simulink model "Model_with_decision"  (R2022a)
settings: Solver=VariableStepAuto  StartTime=0.0  StopTime=1000000  RelTol=1e-3
undefined symbols (not defined in the file): Coefficient_value, Enable_X, Enable_Y, N, s1, s10, s11, s12, s13, s14, s15, s16, s17, s18, s19, s2, s20, s21, s22, s23, s24, s25, s26, s27, s28, s29, s3, s30, s4, s5, s6, s7, s8, s9
libraries: simulink x35
(part 5 of 5)

== system Model_with_decision/Pbit_2/EN=1 Block ==
  note: this is boolean
  note: threshold is subtracted from the sum of total input and random value to implement > 1 comparison
  IN : Inport
  Action Port : ActionPort  ActionPortLabel=if(u1 > 0)
  Add : Sum
  Add1 : Sum
  Compare To Constant : simulink/Logic and Bit Operations/Compare To Constant  relop=>  const=1  OutDataTypeStr=boolean
  Constant : Constant  Value=-1
  Constant1 : Constant
  Constant2 : Constant
  Divide : Product  Inputs=*/
  Math Function : Math
  Product : Product
  Uniform Random Number : UniformRandomNumber  Minimum=0  Seed=s2  SampleTime=1
  OUT : Outport
  wires:
  Add1/1 -> Divide/2
  Constant2/1 -> Divide/1
  Math Function/1 -> Add1/1
  Product/1 -> Math Function/1
  Constant1/1 -> Add1/2
  Constant/1 -> Product/2
  Divide/1 -> Add/1
  IN/1 -> Product/1
  Compare To Constant/1 -> OUT/1
  Add/1 -> Compare To Constant/1
  Uniform Random Number/1 -> Add/2

== system Model_with_decision/Pbit_3/EN=0 Block ==
  IN : Inport
  Action Port : ActionPort  ActionPortLabel=else
  Out1 : Outport
  wires:
  IN/1 -> Out1/1

== system Model_with_decision/Pbit_3/EN=1 Block ==
  note: threshold is subtracted from the sum of total input and random value to implement > 1 comparison
  note: this is boolean
  IN : Inport
  Action Port : ActionPort  ActionPortLabel=if(u1 > 0)
  Add : Sum
  Add1 : Sum
  Compare To Constant : simulink/Logic and Bit Operations/Compare To Constant  relop=>  const=1  OutDataTypeStr=boolean
  Constant : Constant  Value=-1
  Constant1 : Constant
  Constant2 : Constant
  Divide : Product  Inputs=*/
  Math Function : Math
  Product : Product
  Uniform Random Number : UniformRandomNumber  Minimum=0  Seed=s3  SampleTime=1
  OUT : Outport
  wires:
  Uniform Random Number/1 -> Add/2
  Add/1 -> Compare To Constant/1
  Compare To Constant/1 -> OUT/1
  IN/1 -> Product/1
  Divide/1 -> Add/1
  Constant/1 -> Product/2
  Constant1/1 -> Add1/2
  Product/1 -> Math Function/1
  Math Function/1 -> Add1/1
  Constant2/1 -> Divide/1
  Add1/1 -> Divide/2

== system Model_with_decision/Pbit_4/EN=0 Block ==
  IN : Inport
  Action Port : ActionPort  ActionPortLabel=else
  Out1 : Outport
  wires:
  IN/1 -> Out1/1

== system Model_with_decision/Pbit_4/EN=1 Block ==
  note: threshold is subtracted from the sum of total input and random value to implement > 1 comparison
  note: this is boolean
  IN : Inport
  Action Port : ActionPort  ActionPortLabel=if(u1 > 0)
  Add : Sum
  Add1 : Sum
  Compare To Constant : simulink/Logic and Bit Operations/Compare To Constant  relop=>  const=1  OutDataTypeStr=boolean
  Constant : Constant  Value=-1
  Constant1 : Constant
  Constant2 : Constant
  Divide : Product  Inputs=*/
  Math Function : Math
  Product : Product
  Uniform Random Number : UniformRandomNumber  Minimum=0  Seed=s4  SampleTime=1
  OUT : Outport
  wires:
  Uniform Random Number/1 -> Add/2
  Add/1 -> Compare To Constant/1
  Compare To Constant/1 -> OUT/1
  IN/1 -> Product/1
  Divide/1 -> Add/1
  Constant/1 -> Product/2
  Constant1/1 -> Add1/2
  Product/1 -> Math Function/1
  Math Function/1 -> Add1/1
  Constant2/1 -> Divide/1
  Add1/1 -> Divide/2

== system Model_with_decision/Pbit_5/EN=0 Block ==
  IN : Inport
  Action Port : ActionPort  ActionPortLabel=else
  Out1 : Outport
  wires:
  IN/1 -> Out1/1

== system Model_with_decision/Pbit_5/EN=1 Block ==
  note: this is boolean
  note: threshold is subtracted from the sum of total input and random value to implement > 1 comparison
  IN : Inport
  Action Port : ActionPort  ActionPortLabel=if(u1 > 0)
  Add : Sum
  Add1 : Sum
  Compare To Constant : simulink/Logic and Bit Operations/Compare To Constant  relop=>  const=1  OutDataTypeStr=boolean
  Constant : Constant  Value=-1
  Constant1 : Constant
  Constant2 : Constant
  Divide : Product  Inputs=*/
  Math Function : Math
  Product : Product
  Uniform Random Number : UniformRandomNumber  Minimum=0  Seed=s5  SampleTime=1
  OUT : Outport
  wires:
  Add1/1 -> Divide/2
  Constant2/1 -> Divide/1
  Math Function/1 -> Add1/1
  Product/1 -> Math Function/1
  Constant1/1 -> Add1/2
  Constant/1 -> Product/2
  Divide/1 -> Add/1
  IN/1 -> Product/1
  Compare To Constant/1 -> OUT/1
  Add/1 -> Compare To Constant/1
  Uniform Random Number/1 -> Add/2

== system Model_with_decision/Pbit_6/EN=0 Block ==
  IN : Inport
  Action Port : ActionPort  ActionPortLabel=else
  Out1 : Outport
  wires:
  IN/1 -> Out1/1

== system Model_with_decision/Pbit_6/EN=1 Block ==
  note: this is boolean
  note: threshold is subtracted from the sum of total input and random value to implement > 1 comparison
  IN : Inport
  Action Port : ActionPort  ActionPortLabel=if(u1 > 0)
  Add : Sum
  Add1 : Sum
  Compare To Constant : simulink/Logic and Bit Operations/Compare To Constant  relop=>  const=1  OutDataTypeStr=boolean
  Constant : Constant  Value=-1
  Constant1 : Constant
  Constant2 : Constant
  Divide : Product  Inputs=*/
  Math Function : Math
  Product : Product
  Uniform Random Number : UniformRandomNumber  Minimum=0  Seed=s6  SampleTime=1
  OUT : Outport
  wires:
  Add1/1 -> Divide/2
  Constant2/1 -> Divide/1
  Math Function/1 -> Add1/1
  Product/1 -> Math Function/1
  Constant1/1 -> Add1/2
  Constant/1 -> Product/2
  Divide/1 -> Add/1
  IN/1 -> Product/1
  Compare To Constant/1 -> OUT/1
  Add/1 -> Compare To Constant/1
  Uniform Random Number/1 -> Add/2

== system Model_with_decision/Pbit_7/EN=0 Block ==
  IN : Inport
  Action Port : ActionPort  ActionPortLabel=else
  Out1 : Outport
  wires:
  IN/1 -> Out1/1

== system Model_with_decision/Pbit_7/EN=1 Block ==
  note: this is boolean
  note: threshold is subtracted from the sum of total input and random value to implement > 1 comparison
  IN : Inport
  Action Port : ActionPort  ActionPortLabel=if(u1 > 0)
  Add : Sum
  Add1 : Sum
  Compare To Constant : simulink/Logic and Bit Operations/Compare To Constant  relop=>  const=1  OutDataTypeStr=boolean
  Constant : Constant  Value=-1
  Constant1 : Constant
  Constant2 : Constant
  Divide : Product  Inputs=*/
  Math Function : Math
  Product : Product
  Uniform Random Number : UniformRandomNumber  Minimum=0  Seed=s7  SampleTime=1
  OUT : Outport
  wires:
  Add1/1 -> Divide/2
  Constant2/1 -> Divide/1
  Math Function/1 -> Add1/1
  Product/1 -> Math Function/1
  Constant1/1 -> Add1/2
  Constant/1 -> Product/2
  Divide/1 -> Add/1
  IN/1 -> Product/1
  Compare To Constant/1 -> OUT/1
  Add/1 -> Compare To Constant/1
  Uniform Random Number/1 -> Add/2

== system Model_with_decision/Pbit_8/EN=0 Block ==
  IN : Inport
  Action Port : ActionPort  ActionPortLabel=else
  Out1 : Outport
  wires:
  IN/1 -> Out1/1

== system Model_with_decision/Pbit_8/EN=1 Block ==
  note: threshold is subtracted from the sum of total input and random value to implement > 1 comparison
  note: this is boolean
  IN : Inport
  Action Port : ActionPort  ActionPortLabel=if(u1 > 0)
  Add : Sum
  Add1 : Sum
  Compare To Constant : simulink/Logic and Bit Operations/Compare To Constant  relop=>  const=1  OutDataTypeStr=boolean
  Constant : Constant  Value=-1
  Constant1 : Constant
  Constant2 : Constant
  Divide : Product  Inputs=*/
  Math Function : Math
  Product : Product
  Uniform Random Number : UniformRandomNumber  Minimum=0  Seed=s8  SampleTime=1
  OUT : Outport
  wires:
  Uniform Random Number/1 -> Add/2
  Add/1 -> Compare To Constant/1
  Compare To Constant/1 -> OUT/1
  IN/1 -> Product/1
  Divide/1 -> Add/1
  Constant/1 -> Product/2
  Constant1/1 -> Add1/2
  Product/1 -> Math Function/1
  Math Function/1 -> Add1/1
  Constant2/1 -> Divide/1
  Add1/1 -> Divide/2

== system Model_with_decision/Pbit_9/EN=0 Block ==
  IN : Inport
  Action Port : ActionPort  ActionPortLabel=else
  Out1 : Outport
  wires:
  IN/1 -> Out1/1

== system Model_with_decision/Pbit_9/EN=1 Block ==
  note: threshold is subtracted from the sum of total input and random value to implement > 1 comparison
  note: this is boolean
  IN : Inport
  Action Port : ActionPort  ActionPortLabel=if(u1 > 0)
  Add : Sum
  Add1 : Sum
  Compare To Constant : simulink/Logic and Bit Operations/Compare To Constant  relop=>  const=1  OutDataTypeStr=boolean
  Constant : Constant  Value=-1
  Constant1 : Constant
  Constant2 : Constant
  Divide : Product  Inputs=*/
  Math Function : Math
  Product : Product
  Uniform Random Number : UniformRandomNumber  Minimum=0  Seed=s9  SampleTime=1
  OUT : Outport
  wires:
  Uniform Random Number/1 -> Add/2
  Add/1 -> Compare To Constant/1
  Compare To Constant/1 -> OUT/1
  IN/1 -> Product/1
  Divide/1 -> Add/1
  Constant/1 -> Product/2
  Constant1/1 -> Add1/2
  Product/1 -> Math Function/1
  Math Function/1 -> Add1/1
  Constant2/1 -> Divide/1
  Add1/1 -> Divide/2

== system Model_with_decision/Pbit_Y_1/EN=0 Block ==
  IN : Inport
  Action Port : ActionPort  ActionPortLabel=else
  Out1 : Outport
  wires:
  IN/1 -> Out1/1

== system Model_with_decision/Pbit_Y_1/EN=1 Block ==
  note: this is boolean
  note: threshold is subtracted from the sum of total input and random value to implement > 1 comparison
  IN : Inport
  Action Port : ActionPort  ActionPortLabel=if(u1 > 0)
  Add : Sum
  Add1 : Sum
  Compare To Constant : simulink/Logic and Bit Operations/Compare To Constant  relop=>  const=1  OutDataTypeStr=boolean
  Constant : Constant  Value=-1
  Constant1 : Constant
  Constant2 : Constant
  Divide : Product  Inputs=*/
  Math Function : Math
  Product : Product
  Uniform Random Number : UniformRandomNumber  Minimum=0  Seed=s16  SampleTime=1
  OUT : Outport
  wires:
  Add1/1 -> Divide/2
  Constant2/1 -> Divide/1
  Math Function/1 -> Add1/1
  Product/1 -> Math Function/1
  Constant1/1 -> Add1/2
  Constant/1 -> Product/2
  Divide/1 -> Add/1
  IN/1 -> Product/1
  Compare To Constant/1 -> OUT/1
  Add/1 -> Compare To Constant/1
  Uniform Random Number/1 -> Add/2

== system Model_with_decision/Pbit_Y_10/EN=0 Block ==
  IN : Inport
  Action Port : ActionPort  ActionPortLabel=else
  Out1 : Outport
  wires:
  IN/1 -> Out1/1

== system Model_with_decision/Pbit_Y_10/EN=1 Block ==
  note: this is boolean
  note: threshold is subtracted from the sum of total input and random value to implement > 1 comparison
  IN : Inport
  Action Port : ActionPort  ActionPortLabel=if(u1 > 0)
  Add : Sum
  Add1 : Sum
  Compare To Constant : simulink/Logic and Bit Operations/Compare To Constant  relop=>  const=1  OutDataTypeStr=boolean
  Constant : Constant  Value=-1
  Constant1 : Constant
  Constant2 : Constant
  Divide : Product  Inputs=*/
  Math Function : Math
  Product : Product
  Uniform Random Number : UniformRandomNumber  Minimum=0  Seed=s25  SampleTime=1
  OUT : Outport
  wires:
  Add1/1 -> Divide/2
  Constant2/1 -> Divide/1
  Math Function/1 -> Add1/1
  Product/1 -> Math Function/1
  Constant1/1 -> Add1/2
  Constant/1 -> Product/2
  Divide/1 -> Add/1
  IN/1 -> Product/1
  Compare To Constant/1 -> OUT/1
  Add/1 -> Compare To Constant/1
  Uniform Random Number/1 -> Add/2

== system Model_with_decision/Pbit_Y_11/EN=0 Block ==
  IN : Inport
  Action Port : ActionPort  ActionPortLabel=else
  Out1 : Outport
  wires:
  IN/1 -> Out1/1

== system Model_with_decision/Pbit_Y_11/EN=1 Block ==
  note: this is boolean
  note: threshold is subtracted from the sum of total input and random value to implement > 1 comparison
  IN : Inport
  Action Port : ActionPort  ActionPortLabel=if(u1 > 0)
  Add : Sum
  Add1 : Sum
  Compare To Constant : simulink/Logic and Bit Operations/Compare To Constant  relop=>  const=1  OutDataTypeStr=boolean
  Constant : Constant  Value=-1
  Constant1 : Constant
  Constant2 : Constant
  Divide : Product  Inputs=*/
  Math Function : Math
  Product : Product
  Uniform Random Number : UniformRandomNumber  Minimum=0  Seed=s26  SampleTime=1
  OUT : Outport
  wires:
  Add1/1 -> Divide/2
  Constant2/1 -> Divide/1
  Math Function/1 -> Add1/1
  Product/1 -> Math Function/1
  Constant1/1 -> Add1/2
  Constant/1 -> Product/2
  Divide/1 -> Add/1
  IN/1 -> Product/1
  Compare To Constant/1 -> OUT/1
  Add/1 -> Compare To Constant/1
  Uniform Random Number/1 -> Add/2

== system Model_with_decision/Pbit_Y_12/EN=0 Block ==
  IN : Inport
  Action Port : ActionPort  ActionPortLabel=else
  Out1 : Outport
  wires:
  IN/1 -> Out1/1

== system Model_with_decision/Pbit_Y_12/EN=1 Block ==
  note: this is boolean
  note: threshold is subtracted from the sum of total input and random value to implement > 1 comparison
  IN : Inport
  Action Port : ActionPort  ActionPortLabel=if(u1 > 0)
  Add : Sum
  Add1 : Sum
  Compare To Constant : simulink/Logic and Bit Operations/Compare To Constant  relop=>  const=1  OutDataTypeStr=boolean
  Constant : Constant  Value=-1
  Constant1 : Constant
  Constant2 : Constant
  Divide : Product  Inputs=*/
  Math Function : Math
  Product : Product
  Uniform Random Number : UniformRandomNumber  Minimum=0  Seed=s27  SampleTime=1
  OUT : Outport
  wires:
  Add1/1 -> Divide/2
  Constant2/1 -> Divide/1
  Math Function/1 -> Add1/1
  Product/1 -> Math Function/1
  Constant1/1 -> Add1/2
  Constant/1 -> Product/2
  Divide/1 -> Add/1
  IN/1 -> Product/1
  Compare To Constant/1 -> OUT/1
  Add/1 -> Compare To Constant/1
  Uniform Random Number/1 -> Add/2

== system Model_with_decision/Pbit_Y_13/EN=0 Block ==
  IN : Inport
  Action Port : ActionPort  ActionPortLabel=else
  Out1 : Outport
  wires:
  IN/1 -> Out1/1

== system Model_with_decision/Pbit_Y_13/EN=1 Block ==
  note: threshold is subtracted from the sum of total input and random value to implement > 1 comparison
  note: this is boolean
  IN : Inport
  Action Port : ActionPort  ActionPortLabel=if(u1 > 0)
  Add : Sum
  Add1 : Sum
  Compare To Constant : simulink/Logic and Bit Operations/Compare To Constant  relop=>  const=1  OutDataTypeStr=boolean
  Constant : Constant  Value=-1
  Constant1 : Constant
  Constant2 : Constant
  Divide : Product  Inputs=*/
  Math Function : Math
  Product : Product
  Uniform Random Number : UniformRandomNumber  Minimum=0  Seed=s28  SampleTime=1
  OUT : Outport
  wires:
  Uniform Random Number/1 -> Add/2
  Add/1 -> Compare To Constant/1
  Compare To Constant/1 -> OUT/1
  IN/1 -> Product/1
  Divide/1 -> Add/1
  Constant/1 -> Product/2
  Constant1/1 -> Add1/2
  Product/1 -> Math Function/1
  Math Function/1 -> Add1/1
  Constant2/1 -> Divide/1
  Add1/1 -> Divide/2

== system Model_with_decision/Pbit_Y_14/EN=0 Block ==
  IN : Inport
  Action Port : ActionPort  ActionPortLabel=else
  Out1 : Outport
  wires:
  IN/1 -> Out1/1

== system Model_with_decision/Pbit_Y_14/EN=1 Block ==
  note: threshold is subtracted from the sum of total input and random value to implement > 1 comparison
  note: this is boolean
  IN : Inport
  Action Port : ActionPort  ActionPortLabel=if(u1 > 0)
  Add : Sum
  Add1 : Sum
  Compare To Constant : simulink/Logic and Bit Operations/Compare To Constant  relop=>  const=1  OutDataTypeStr=boolean
  Constant : Constant  Value=-1
  Constant1 : Constant
  Constant2 : Constant
  Divide : Product  Inputs=*/
  Math Function : Math
  Product : Product
  Uniform Random Number : UniformRandomNumber  Minimum=0  Seed=s29  SampleTime=1
  OUT : Outport
  wires:
  Uniform Random Number/1 -> Add/2
  Add/1 -> Compare To Constant/1
  Compare To Constant/1 -> OUT/1
  IN/1 -> Product/1
  Divide/1 -> Add/1
  Constant/1 -> Product/2
  Constant1/1 -> Add1/2
  Product/1 -> Math Function/1
  Math Function/1 -> Add1/1
  Constant2/1 -> Divide/1
  Add1/1 -> Divide/2

== system Model_with_decision/Pbit_Y_15/EN=0 Block ==
  IN : Inport
  Action Port : ActionPort  ActionPortLabel=else
  Out1 : Outport
  wires:
  IN/1 -> Out1/1

== system Model_with_decision/Pbit_Y_15/EN=1 Block ==
  note: threshold is subtracted from the sum of total input and random value to implement > 1 comparison
  note: this is boolean
  IN : Inport
  Action Port : ActionPort  ActionPortLabel=if(u1 > 0)
  Add : Sum
  Add1 : Sum
  Compare To Constant : simulink/Logic and Bit Operations/Compare To Constant  relop=>  const=1  OutDataTypeStr=boolean
  Constant : Constant  Value=-1
  Constant1 : Constant
  Constant2 : Constant
  Divide : Product  Inputs=*/
  Math Function : Math
  Product : Product
  Uniform Random Number : UniformRandomNumber  Minimum=0  Seed=s30  SampleTime=1
  OUT : Outport
  wires:
  Uniform Random Number/1 -> Add/2
  Add/1 -> Compare To Constant/1
  Compare To Constant/1 -> OUT/1
  IN/1 -> Product/1
  Divide/1 -> Add/1
  Constant/1 -> Product/2
  Constant1/1 -> Add1/2
  Product/1 -> Math Function/1
  Math Function/1 -> Add1/1
  Constant2/1 -> Divide/1
  Add1/1 -> Divide/2

== system Model_with_decision/Pbit_Y_2/EN=0 Block ==
  IN : Inport
  Action Port : ActionPort  ActionPortLabel=else
  Out1 : Outport
  wires:
  IN/1 -> Out1/1

== system Model_with_decision/Pbit_Y_2/EN=1 Block ==
  note: this is boolean
  note: threshold is subtracted from the sum of total input and random value to implement > 1 comparison
  IN : Inport
  Action Port : ActionPort  ActionPortLabel=if(u1 > 0)
  Add : Sum
  Add1 : Sum
  Compare To Constant : simulink/Logic and Bit Operations/Compare To Constant  relop=>  const=1  OutDataTypeStr=boolean
  Constant : Constant  Value=-1
  Constant1 : Constant
  Constant2 : Constant
  Divide : Product  Inputs=*/
  Math Function : Math
  Product : Product
  Uniform Random Number : UniformRandomNumber  Minimum=0  Seed=s17  SampleTime=1
  OUT : Outport
  wires:
  Add1/1 -> Divide/2
  Constant2/1 -> Divide/1
  Math Function/1 -> Add1/1
  Product/1 -> Math Function/1
  Constant1/1 -> Add1/2
  Constant/1 -> Product/2
  Divide/1 -> Add/1
  IN/1 -> Product/1
  Compare To Constant/1 -> OUT/1
  Add/1 -> Compare To Constant/1
  Uniform Random Number/1 -> Add/2

== system Model_with_decision/Pbit_Y_3/EN=0 Block ==
  IN : Inport
  Action Port : ActionPort  ActionPortLabel=else
  Out1 : Outport
  wires:
  IN/1 -> Out1/1

== system Model_with_decision/Pbit_Y_3/EN=1 Block ==
  note: threshold is subtracted from the sum of total input and random value to implement > 1 comparison
  note: this is boolean
  IN : Inport
  Action Port : ActionPort  ActionPortLabel=if(u1 > 0)
  Add : Sum
  Add1 : Sum
  Compare To Constant : simulink/Logic and Bit Operations/Compare To Constant  relop=>  const=1  OutDataTypeStr=boolean
  Constant : Constant  Value=-1
  Constant1 : Constant
  Constant2 : Constant
  Divide : Product  Inputs=*/
  Math Function : Math
  Product : Product
  Uniform Random Number : UniformRandomNumber  Minimum=0  Seed=s18  SampleTime=1
  OUT : Outport
  wires:
  Uniform Random Number/1 -> Add/2
  Add/1 -> Compare To Constant/1
  Compare To Constant/1 -> OUT/1
  IN/1 -> Product/1
  Divide/1 -> Add/1
  Constant/1 -> Product/2
  Constant1/1 -> Add1/2
  Product/1 -> Math Function/1
  Math Function/1 -> Add1/1
  Constant2/1 -> Divide/1
  Add1/1 -> Divide/2

== system Model_with_decision/Pbit_Y_4/EN=0 Block ==
  IN : Inport
  Action Port : ActionPort  ActionPortLabel=else
  Out1 : Outport
  wires:
  IN/1 -> Out1/1

== system Model_with_decision/Pbit_Y_4/EN=1 Block ==
  note: threshold is subtracted from the sum of total input and random value to implement > 1 comparison
  note: this is boolean
  IN : Inport
  Action Port : ActionPort  ActionPortLabel=if(u1 > 0)
  Add : Sum
  Add1 : Sum
  Compare To Constant : simulink/Logic and Bit Operations/Compare To Constant  relop=>  const=1  OutDataTypeStr=boolean
  Constant : Constant  Value=-1
  Constant1 : Constant
  Constant2 : Constant
  Divide : Product  Inputs=*/
  Math Function : Math
  Product : Product
  Uniform Random Number : UniformRandomNumber  Minimum=0  Seed=s19  SampleTime=1
  OUT : Outport
  wires:
  Uniform Random Number/1 -> Add/2
  Add/1 -> Compare To Constant/1
  Compare To Constant/1 -> OUT/1
  IN/1 -> Product/1
  Divide/1 -> Add/1
  Constant/1 -> Product/2
  Constant1/1 -> Add1/2
  Product/1 -> Math Function/1
  Math Function/1 -> Add1/1
  Constant2/1 -> Divide/1
  Add1/1 -> Divide/2

== system Model_with_decision/Pbit_Y_5/EN=0 Block ==
  IN : Inport
  Action Port : ActionPort  ActionPortLabel=else
  Out1 : Outport
  wires:
  IN/1 -> Out1/1

== system Model_with_decision/Pbit_Y_5/EN=1 Block ==
  note: this is boolean
  note: threshold is subtracted from the sum of total input and random value to implement > 1 comparison
  IN : Inport
  Action Port : ActionPort  ActionPortLabel=if(u1 > 0)
  Add : Sum
  Add1 : Sum
  Compare To Constant : simulink/Logic and Bit Operations/Compare To Constant  relop=>  const=1  OutDataTypeStr=boolean
  Constant : Constant  Value=-1
  Constant1 : Constant
  Constant2 : Constant
  Divide : Product  Inputs=*/
  Math Function : Math
  Product : Product
  Uniform Random Number : UniformRandomNumber  Minimum=0  Seed=s20  SampleTime=1
  OUT : Outport
  wires:
  Add1/1 -> Divide/2
  Constant2/1 -> Divide/1
  Math Function/1 -> Add1/1
  Product/1 -> Math Function/1
  Constant1/1 -> Add1/2
  Constant/1 -> Product/2
  Divide/1 -> Add/1
  IN/1 -> Product/1
  Compare To Constant/1 -> OUT/1
  Add/1 -> Compare To Constant/1
  Uniform Random Number/1 -> Add/2

== system Model_with_decision/Pbit_Y_6/EN=0 Block ==
  IN : Inport
  Action Port : ActionPort  ActionPortLabel=else
  Out1 : Outport
  wires:
  IN/1 -> Out1/1

== system Model_with_decision/Pbit_Y_6/EN=1 Block ==
  note: this is boolean
  note: threshold is subtracted from the sum of total input and random value to implement > 1 comparison
  IN : Inport
  Action Port : ActionPort  ActionPortLabel=if(u1 > 0)
  Add : Sum
  Add1 : Sum
  Compare To Constant : simulink/Logic and Bit Operations/Compare To Constant  relop=>  const=1  OutDataTypeStr=boolean
  Constant : Constant  Value=-1
  Constant1 : Constant
  Constant2 : Constant
  Divide : Product  Inputs=*/
  Math Function : Math
  Product : Product
  Uniform Random Number : UniformRandomNumber  Minimum=0  Seed=s21  SampleTime=1
  OUT : Outport
  wires:
  Add1/1 -> Divide/2
  Constant2/1 -> Divide/1
  Math Function/1 -> Add1/1
  Product/1 -> Math Function/1
  Constant1/1 -> Add1/2
  Constant/1 -> Product/2
  Divide/1 -> Add/1
  IN/1 -> Product/1
  Compare To Constant/1 -> OUT/1
  Add/1 -> Compare To Constant/1
  Uniform Random Number/1 -> Add/2

== system Model_with_decision/Pbit_Y_7/EN=0 Block ==
  IN : Inport
  Action Port : ActionPort  ActionPortLabel=else
  Out1 : Outport
  wires:
  IN/1 -> Out1/1

== system Model_with_decision/Pbit_Y_7/EN=1 Block ==
  note: this is boolean
  note: threshold is subtracted from the sum of total input and random value to implement > 1 comparison
  IN : Inport
  Action Port : ActionPort  ActionPortLabel=if(u1 > 0)
  Add : Sum
  Add1 : Sum
  Compare To Constant : simulink/Logic and Bit Operations/Compare To Constant  relop=>  const=1  OutDataTypeStr=boolean
  Constant : Constant  Value=-1
  Constant1 : Constant
  Constant2 : Constant
  Divide : Product  Inputs=*/
  Math Function : Math
  Product : Product
  Uniform Random Number : UniformRandomNumber  Minimum=0  Seed=s22  SampleTime=1
  OUT : Outport
  wires:
  Add1/1 -> Divide/2
  Constant2/1 -> Divide/1
  Math Function/1 -> Add1/1
  Product/1 -> Math Function/1
  Constant1/1 -> Add1/2
  Constant/1 -> Product/2
  Divide/1 -> Add/1
  IN/1 -> Product/1
  Compare To Constant/1 -> OUT/1
  Add/1 -> Compare To Constant/1
  Uniform Random Number/1 -> Add/2

== system Model_with_decision/Pbit_Y_8/EN=0 Block ==
  IN : Inport
  Action Port : ActionPort  ActionPortLabel=else
  Out1 : Outport
  wires:
  IN/1 -> Out1/1

== system Model_with_decision/Pbit_Y_8/EN=1 Block ==
  note: threshold is subtracted from the sum of total input and random value to implement > 1 comparison
  note: this is boolean
  IN : Inport
  Action Port : ActionPort  ActionPortLabel=if(u1 > 0)
  Add : Sum
  Add1 : Sum
  Compare To Constant : simulink/Logic and Bit Operations/Compare To Constant  relop=>  const=1  OutDataTypeStr=boolean
  Constant : Constant  Value=-1
  Constant1 : Constant
  Constant2 : Constant
  Divide : Product  Inputs=*/
  Math Function : Math
  Product : Product
  Uniform Random Number : UniformRandomNumber  Minimum=0  Seed=s23  SampleTime=1
  OUT : Outport
  wires:
  Uniform Random Number/1 -> Add/2
  Add/1 -> Compare To Constant/1
  Compare To Constant/1 -> OUT/1
  IN/1 -> Product/1
  Divide/1 -> Add/1
  Constant/1 -> Product/2
  Constant1/1 -> Add1/2
  Product/1 -> Math Function/1
  Math Function/1 -> Add1/1
  Constant2/1 -> Divide/1
  Add1/1 -> Divide/2

== system Model_with_decision/Pbit_Y_9/EN=0 Block ==
  IN : Inport
  Action Port : ActionPort  ActionPortLabel=else
  Out1 : Outport
  wires:
  IN/1 -> Out1/1

== system Model_with_decision/Pbit_Y_9/EN=1 Block ==
  note: threshold is subtracted from the sum of total input and random value to implement > 1 comparison
  note: this is boolean
  IN : Inport
  Action Port : ActionPort  ActionPortLabel=if(u1 > 0)
  Add : Sum
  Add1 : Sum
  Compare To Constant : simulink/Logic and Bit Operations/Compare To Constant  relop=>  const=1  OutDataTypeStr=boolean
  Constant : Constant  Value=-1
  Constant1 : Constant
  Constant2 : Constant
  Divide : Product  Inputs=*/
  Math Function : Math
  Product : Product
  Uniform Random Number : UniformRandomNumber  Minimum=0  Seed=s24  SampleTime=1
  OUT : Outport
  wires:
  Uniform Random Number/1 -> Add/2
  Add/1 -> Compare To Constant/1
  Compare To Constant/1 -> OUT/1
  IN/1 -> Product/1
  Divide/1 -> Add/1
  Constant/1 -> Product/2
  Constant1/1 -> Add1/2
  Product/1 -> Math Function/1
  Math Function/1 -> Add1/1
  Constant2/1 -> Divide/1
  Add1/1 -> Divide/2
